simulink model "test"  (Simulink 6.5)
settings: Solver=ode45  StartTime=0.0  StopTime=10.0  RelTol=1e-3
libraries: cdsFilt x5, cdsEpicsOut x2, cdsRfmIO x1, cdsOsc x1, cdsPhase x1
settings Model: Creator=rolf  LastModifiedBy=aivanov  ExtModeAutoUpdateStatusClock=off
settings DebuggingCC: MultiTaskDSMMsg=warning  MultiTaskCondExecSysMsg=none  StrictBusMsg=None
settings RTWCC: IncludeERTFirstTime=on

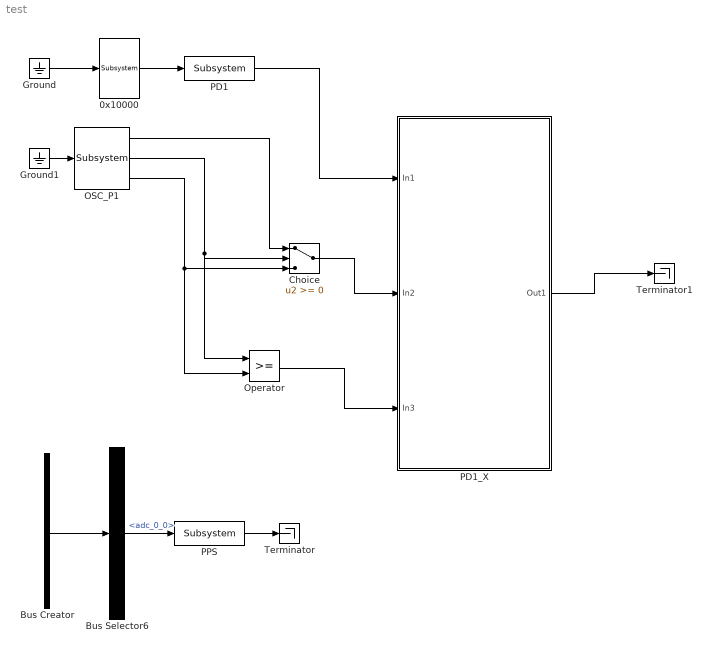
== system test ==
  0x10000 : cdsRfmIO/Subsystem  Tag=cdsRfmIO  Description=VMIC5565 Reflective Memory read/write  SystemSampleTime=-1
      settings: AttributesFormatString=%<Tag>
  Bus Creator : BusCreator  Inputs='adc_0_0','adc_0_1','adc_0_2','adc_0_3','adc_0_4','adc_0_5','adc_0_6','adc_0_7','adc_0_8','adc_0_9','adc_0_10','adc_0_11','adc_0_12','adc_0_13','adc_0_14','adc_0_15','adc_0_16','adc_0_17','adc_0_18','adc_0_19','adc_0_20','adc_0_21','adc_0_22','adc_0_23','adc_0_24','adc_0_25','adc_0_26','adc_0_27','adc_0_28','adc_0_29','adc_0_30','adc_0_31'
  Bus Selector6 : BusSelector  OutputSignals=adc_0_0
  Choice : Switch
  Ground : Ground
  Ground1 : Ground
  OSC_P1 : cdsOsc/Subsystem  Tag=cdsOsc  Description=Oscillator  SystemSampleTime=-1
      settings: AttributesFormatString=%<Tag>
  Operator : RelationalOperator  LogicOutDataTypeMode=Boolean
  PD1 : cdsFilt/Subsystem  Tag=cdsFilt  Description=|  SystemSampleTime=-1
      | Purpose:                                                                                                                                                                                                                                  
      | Standard CDS IIR filter module.                                                                                                                                                                                                           
      |                                                                                                                                                                                                                                           
      | Operation:                                                                                                                                                                                                                                
      | Consists of 10 second order section IIR filters, plus a ramped gain stage. In FE code, also provides pre-defined test points and excitation channel inputs. The filter coefficients are defined in the LIGO system using the 'foton' tool.
      |                                                                                                                                                                                                                                           
      | Usage:                                                                                                                                                                                                                                    
      | Name the part with the desired filter module name.
      settings: AttributesFormatString=%<Tag>
  PD1_X : Subsystem
  PPS : cdsFilt/Subsystem  Tag=cdsFilt  Description=|  SystemSampleTime=-1
      | Purpose:                                                                                                                                                                                                                                  
      | Standard CDS IIR filter module.                                                                                                                                                                                                           
      |                                                                                                                                                                                                                                           
      | Operation:                                                                                                                                                                                                                                
      | Consists of 10 second order section IIR filters, plus a ramped gain stage. In FE code, also provides pre-defined test points and excitation channel inputs. The filter coefficients are defined in the LIGO system using the 'foton' tool.
      |                                                                                                                                                                                                                                           
      | Usage:                                                                                                                                                                                                                                    
      | Name the part with the desired filter module name.
      settings: AttributesFormatString=%<Tag>
  Terminator : Terminator
  Terminator1 : Terminator
  wires:
  Bus Creator/1 -> Bus Selector6/1
  Ground1/1 -> OSC_P1/1
  Bus Selector6/1 -> PPS/1  "<adc_0_0>"
  PPS/1 -> Terminator/1
  ? -> ?
  ? -> ?
  Ground/1 -> 0x10000/1
  0x10000/1 -> PD1/1
  PD1/1 -> PD1_X/1(In1)
  PD1_X/1(Out1) -> Terminator1/1
  OSC_P1/3 -> Operator/2, Choice/3
  OSC_P1/2 -> Operator/1, Choice/2
  OSC_P1/1 -> Choice/1
  Choice/1 -> PD1_X/2(In2)
  Operator/1 -> PD1_X/3(In3)

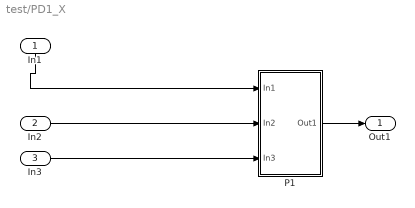
== system test/PD1_X ==
  In1 : Inport  Orientation=down
  In2 : Inport  Port=2
  In3 : Inport  Port=3
  P1 : Subsystem
  Out1 : Outport
  wires:
  In1/1 -> P1/1(In1)
  In2/1 -> P1/2(In2)
  P1/1(Out1) -> Out1/1
  In3/1 -> P1/3(In3)

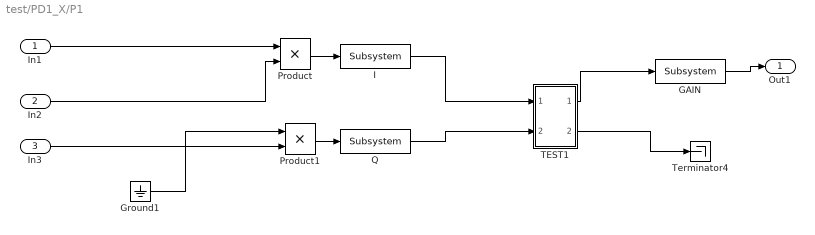
== system test/PD1_X/P1 ==
  In1 : Inport
  In2 : Inport  Port=2
  In3 : Inport  Port=3
  GAIN : cdsFilt/Subsystem  Tag=cdsFilt  Description=|  SystemSampleTime=-1
      | Purpose:                                                                                                                                                                                                                                  
      | Standard CDS IIR filter module.                                                                                                                                                                                                           
      |                                                                                                                                                                                                                                           
      | Operation:                                                                                                                                                                                                                                
      | Consists of 10 second order section IIR filters, plus a ramped gain stage. In FE code, also provides pre-defined test points and excitation channel inputs. The filter coefficients are defined in the LIGO system using the 'foton' tool.
      |                                                                                                                                                                                                                                           
      | Usage:                                                                                                                                                                                                                                    
      | Name the part with the desired filter module name.
      settings: AttributesFormatString=%<Tag>
  Ground1 : Ground
  I : cdsFilt/Subsystem  Tag=cdsFilt  Description=|  SystemSampleTime=-1
      | Purpose:                                                                                                                                                                                                                                  
      | Standard CDS IIR filter module.                                                                                                                                                                                                           
      |                                                                                                                                                                                                                                           
      | Operation:                                                                                                                                                                                                                                
      | Consists of 10 second order section IIR filters, plus a ramped gain stage. In FE code, also provides pre-defined test points and excitation channel inputs. The filter coefficients are defined in the LIGO system using the 'foton' tool.
      |                                                                                                                                                                                                                                           
      | Usage:                                                                                                                                                                                                                                    
      | Name the part with the desired filter module name.
      settings: AttributesFormatString=%<Tag>
  Product : Product  RndMeth=Zero
  Product1 : Product  RndMeth=Zero
  Q : cdsFilt/Subsystem  Tag=cdsFilt  Description=|  SystemSampleTime=-1
      | Purpose:                                                                                                                                                                                                                                  
      | Standard CDS IIR filter module.                                                                                                                                                                                                           
      |                                                                                                                                                                                                                                           
      | Operation:                                                                                                                                                                                                                                
      | Consists of 10 second order section IIR filters, plus a ramped gain stage. In FE code, also provides pre-defined test points and excitation channel inputs. The filter coefficients are defined in the LIGO system using the 'foton' tool.
      |                                                                                                                                                                                                                                           
      | Usage:                                                                                                                                                                                                                                    
      | Name the part with the desired filter module name.
      settings: AttributesFormatString=%<Tag>
  TEST1 : Subsystem
  Terminator4 : Terminator
  Out1 : Outport
  wires:
  TEST1/1(Out1) -> GAIN/1
  Q/1 -> TEST1/2(In2)
  I/1 -> TEST1/1(In1)
  Product/1 -> I/1
  Product1/1 -> Q/1
  GAIN/1 -> Out1/1
  TEST1/2(Out2) -> Terminator4/1
  In1/1 -> Product/1
  In2/1 -> Product/2
  In3/1 -> Product1/2
  Ground1/1 -> Product1/1

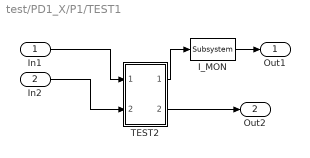
== system test/PD1_X/P1/TEST1 ==
  In1 : Inport
  In2 : Inport  Port=2
  I_MON : cdsEpicsOut/Subsystem  Tag=cdsEpicsOutput  Description=|  SystemSampleTime=-1
      | Purpose:                                          
      | Output a FE signal to an EPICS channel.           
      |                                                   
      | Operation:                                        
      | Takes input value and passes it to EPICS record.  
      |                                                   
      | Usage:                                            
      | Name the part with the desired EPICS rrecord name.
      settings: AttributesFormatString=%<Tag>
  TEST2 : Subsystem
  Out1 : Outport
  Out2 : Outport  Port=2
  wires:
  TEST2/1(Out1) -> I_MON/1
  I_MON/1 -> Out1/1
  In1/1 -> TEST2/1(In1)
  In2/1 -> TEST2/2(In2)
  TEST2/2(Out2) -> Out2/1

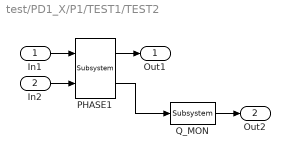
== system test/PD1_X/P1/TEST1/TEST2 ==
  In1 : Inport
  In2 : Inport  Port=2
  PHASE1 : cdsPhase/Subsystem  Tag=cdsPhase  Description=Phase Rotator  SystemSampleTime=-1
      settings: AttributesFormatString=%<Tag>
  Q_MON : cdsEpicsOut/Subsystem  Tag=cdsEpicsOutput  Description=|  SystemSampleTime=-1
      | Purpose:                                          
      | Output a FE signal to an EPICS channel.           
      |                                                   
      | Operation:                                        
      | Takes input value and passes it to EPICS record.  
      |                                                   
      | Usage:                                            
      | Name the part with the desired EPICS rrecord name.
      settings: AttributesFormatString=%<Tag>
  Out1 : Outport
  Out2 : Outport  Port=2
  wires:
  PHASE1/2 -> Q_MON/1
  In1/1 -> PHASE1/1
  PHASE1/1 -> Out1/1
  In2/1 -> PHASE1/2
  Q_MON/1 -> Out2/1
